simulink model "SolarPanelSimplified"  (R2016b)
settings: Solver=VariableStepAuto  StartTime=0.0  StopTime=10.0  RelTol=1e-3
undefined symbols (not defined in the file): vt_panel
libraries: powerlib x10
settings Model: Creator=hp  LastModifiedBy=hp

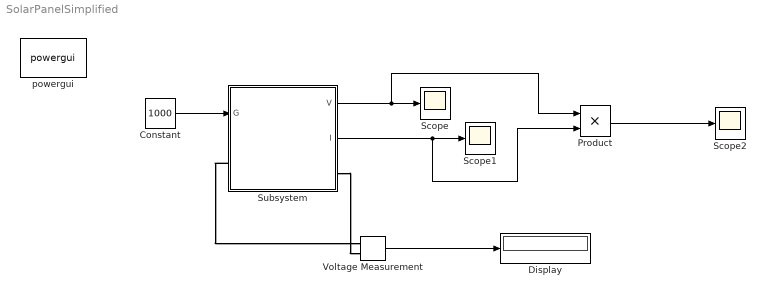
== system SolarPanelSimplified ==
  Constant : Constant  Value=1000
  Display : Display
  Product : Product
  Scope : Scope
  Scope1 : Scope
  Scope2 : Scope
  Subsystem : Subsystem  mask{Ns=0, Np=0}
      mask init:
      | v = 1.5;
      | k = 1.3806e-23;
      | T = 298;
      | q = 1.602e-19;
      | Vt = v*k*T/q;
      | Vt_panel = Vt*Ns;
      | Iph=8;
      | Iph_panel=Iph*Np;
      | Io= 9.845e-7;
      | Io_panel=Io*Np;
      | Rs=0.001;
      | Rs_panel=Rs*Ns/Np;
      | Rsh=142.94;
      | Rsh_panel=Rsh*Ns/Np;
      | G0=1000;
  Voltage Measurement : powerlib/Measurements/Voltage Measurement  PhasorSimulation=off  OutputType=Complex  PSBequivalent=0
  powergui : powerlib/powergui  Priority=1  SimulationMode=Discrete  SolverType=Tustin/Backward Euler (TBE)  SampleTime=50e-6  frequency=60  SPID=off  DisableSnubberDevices=off  DisableRonSwitches=off  DisableVfSwitches=off  SwTol=0  DisplayEquations=off  Interpol=off  ExternalGateDelay=off  methode=off  Ts=10  FunctionMessages=off  echomessages=off  HookPort=off  EnableUseOfTLC=off  x0status=blocks  frequencyindice=60  Pbase=100e6  ErrMax=1e-4  Iterations=50  UnitsV=kV  UnitsW=MW  buscounter=0  RestoreLinks=warning  ResistiveCurrentMeasurement=off  Frange=[0:2:500]  Ylog=off  Xlog=on  ShowGrid=off  save=off  variable=ZData  structure=0  ZoomFFT=off  StartTime=0.0  cycles=1  DisplayStyle=1  fundamental=60  FreqAxis=off  MaxFrequency=1000  frequencyindicesteady=1  RmsSteady=1  display=off
  wires:
  Constant/1 -> Subsystem/1(G)
  Voltage Measurement/1 -> Display/1
  Subsystem/1(V) -> Product/1, Scope/1
  Subsystem/2(I) -> Product/2, Scope1/1
  Product/1 -> Scope2/1
  connections:
  Subsystem/LConn1 -- Voltage Measurement/LConn1
  Subsystem/RConn1 -- Voltage Measurement/LConn2

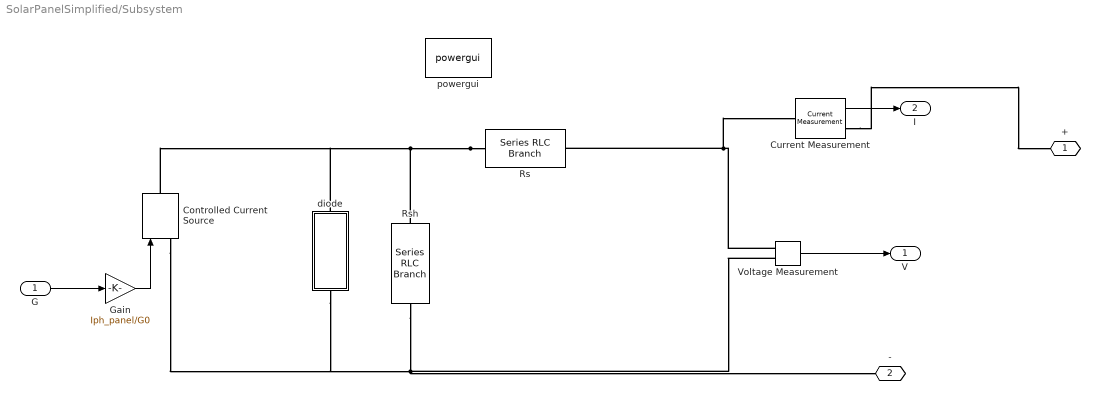
== system SolarPanelSimplified/Subsystem ==
  G : Inport
  Controlled Current Source : powerlib/Electrical Sources/Controlled Current Source  Initialize=on  Source_Type=AC  Amplitude=0  Phase=0  Frequency=0  Measurements=None
  Current Measurement : powerlib/Measurements/Current Measurement  PhasorSimulation=off  OutputType=Complex  PSBequivalent=0
  Gain : Gain  Gain=Iph_panel/G0
  Rs : powerlib/Elements/Series RLC Branch  LConnTagsString=__new0  RConnTagsString=__new0  BranchType=R  Resistance=Rs  Inductance=1e-3  SetiL0=off  InitialCurrent=0  Capacitance=1e-6  Setx0=off  InitialVoltage=0  Measurements=None
  Rsh : powerlib/Elements/Series RLC Branch  LConnTagsString=__new0  RConnTagsString=__new0  BranchType=R  Resistance=Rsh  Inductance=1e-3  SetiL0=off  InitialCurrent=0  Capacitance=1e-6  Setx0=off  InitialVoltage=0  Measurements=None
  Voltage Measurement : powerlib/Measurements/Voltage Measurement  PhasorSimulation=off  OutputType=Complex  PSBequivalent=0
  "diode " : Subsystem
  powergui : powerlib/powergui  Priority=1  SimulationMode=Continuous  SolverType=Tustin/Backward Euler (TBE)  SampleTime=50e-6  frequency=60  SPID=off  DisableSnubberDevices=off  DisableRonSwitches=off  DisableVfSwitches=off  SwTol=0  DisplayEquations=off  Interpol=off  ExternalGateDelay=off  methode=off  Ts=10  FunctionMessages=off  echomessages=off  HookPort=off  EnableUseOfTLC=off  x0status=blocks  frequencyindice=60  Pbase=100e6  ErrMax=1e-4  Iterations=50  UnitsV=kV  UnitsW=MW  buscounter=0  RestoreLinks=warning  ResistiveCurrentMeasurement=off  Frange=[0:2:500]  Ylog=off  Xlog=on  ShowGrid=off  save=off  variable=ZData  structure=0  ZoomFFT=off  StartTime=0.0  cycles=1  DisplayStyle=1  fundamental=60  FreqAxis=off  MaxFrequency=1000  frequencyindicesteady=1  RmsSteady=1  display=off
  + : PMIOPort  Port=1  Side=Left
  - : PMIOPort  Port=2  Side=Right
  V : Outport
  I : Outport  Port=2
  wires:
  G/1 -> Gain/1
  Gain/1 -> Controlled Current Source/1
  Voltage Measurement/1 -> V/1
  Current Measurement/1 -> I/1
  connections:
  Rs/LConn1 -- Rsh/LConn1 -- "diode "/LConn1 -- Controlled Current Source/RConn1
  Rsh/RConn1 -- Voltage Measurement/LConn2 -- -/RConn1 -- Controlled Current Source/LConn1 -- "diode "/RConn1
  Voltage Measurement/LConn1 -- Current Measurement/LConn1 -- Rs/RConn1
  Current Measurement/RConn1 -- +/RConn1

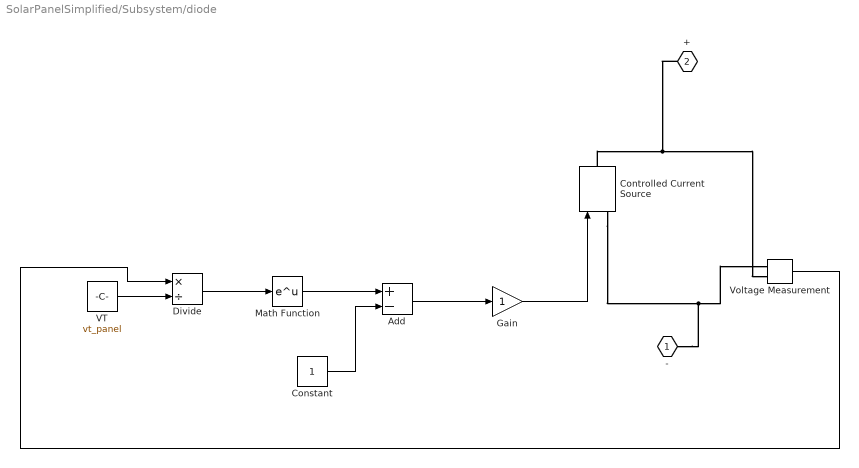
== system SolarPanelSimplified/Subsystem/diode  ==
  Add : Sum  Inputs=+-
  Constant : Constant
  Controlled Current Source : powerlib/Electrical Sources/Controlled Current Source  Initialize=on  Source_Type=AC  Amplitude=0  Phase=0  Frequency=0  Measurements=None
  Divide : Product  Inputs=*/
  Gain : Gain
  Math Function : Math  SaturateOnIntegerOverflow=on
  VT : Constant  Value=vt_panel
  Voltage Measurement : powerlib/Measurements/Voltage Measurement  PhasorSimulation=off  OutputType=Complex  PSBequivalent=0
  - : PMIOPort  Port=1  Side=Right
  + : PMIOPort  Port=2  Side=Left
  wires:
  VT/1 -> Divide/2
  Divide/1 -> Math Function/1
  Math Function/1 -> Add/1
  Add/1 -> Gain/1
  Gain/1 -> Controlled Current Source/1
  Constant/1 -> Add/2
  Voltage Measurement/1 -> Divide/1
  connections:
  +/RConn1 -- Controlled Current Source/RConn1 -- Voltage Measurement/LConn2
  -/RConn1 -- Controlled Current Source/LConn1 -- Voltage Measurement/LConn1
